simulink model "DPT"  (R2023a)
settings: Solver=VariableStepAuto  StartTime=0.0  StopTime=10.0  RelTol=1e-3
values from neighbouring files (symbols this model uses):
  J_a = 3.6 * 10^(-6)    (= 3.6e-06)    [main.m]
  k_m = P_nom / (N_nom * I_a)    (= 0.0014)    [main.m]
  k_w = (U_a - R_a * I_a)/ w_nom    (= 0.0264197205533)    [main.m]
  L_a = 0.1*((J_a * (R_a)^2)/(k_m * k_w))    (= 0.0429224827611)    [main.m]
  R_a = 2.1    [main.m]
libraries: simulink x1, SignalEditorBlockLib x1
settings Model: Creator=ycheb  LastModifiedBy=ycheb

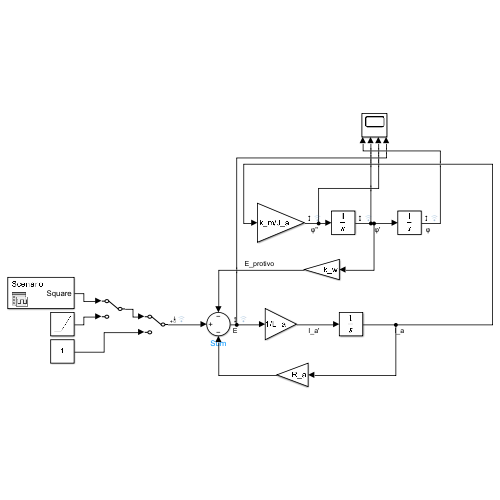
[thumbnail: Simulink's stored preview of the top-level diagram]
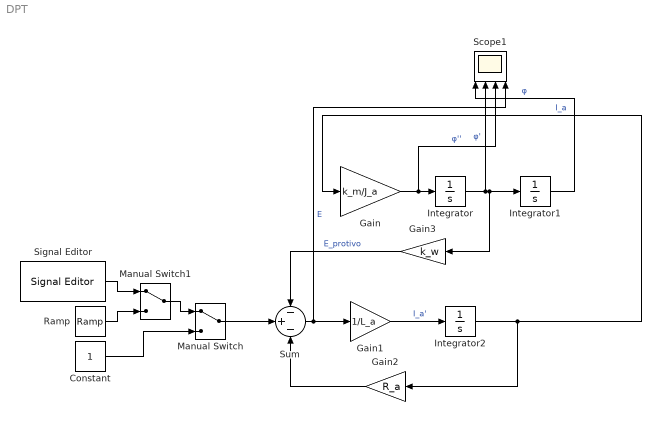
== system DPT ==
  Constant : Constant
  Gain : Gain  Gain=k_m/J_a
  Gain1 : Gain  Gain=1/L_a
  Gain2 : Gain  Gain=R_a
  Gain3 : Gain  Gain=k_w
  Integrator : Integrator
  Integrator1 : Integrator
  Integrator2 : Integrator
  Manual Switch : ManualSwitch
  Manual Switch1 : ManualSwitch
  Ramp : simulink/Sources/Ramp  slope=1  start=0  InitialOutput=0
  Scope1 : Scope  NumInputPorts=4
  Signal Editor : SignalEditorBlockLib/Signal Editor  FileName=Square_signal.mat  ActiveScenario=Scenario  ActiveSignal=Square  IsBus=off  OutputBusObjectStr=Bus: BusObject  SampleTime=0  Interpolate=off  ZeroCross=off  OutputAfterFinalValue=Setting to zero  Unit=inherit  PreserveSignalName=on  ApplySigPropsToAllScenarios=on
  Sum : Sum  Inputs=-+-
  wires:
  Integrator/1 -> Integrator1/1, Gain3/1, Scope1/2  "φ'"
  Gain/1 -> Scope1/3, Integrator/1  "φ''"
  Gain1/1 -> Integrator2/1  "I_a'"
  Integrator2/1 -> Gain/1, Gain2/1  "I_a"
  Sum/1 -> Scope1/4, Gain1/1  "E"
  Gain2/1 -> Sum/3
  Gain3/1 -> Sum/1  "E_protivo"
  Integrator1/1 -> Scope1/1  "φ"
  Manual Switch/1 -> Sum/2
  Constant/1 -> Manual Switch/2
  Ramp/1 -> Manual Switch1/2
  Signal Editor/1 -> Manual Switch1/1
  Manual Switch1/1 -> Manual Switch/1
